simulink model "CRC"  (R2021a)
settings: Solver=ode45  StartTime=0.0  StopTime=10  RelTol=1e-3  EnableMultiTasking=on
model workspace (MAT data in the model file):
  frame_length = -4
undefined symbols (not defined in the file): CRC_degree
libraries: simulink x3, commcrc2 x2, dspswit3 x1
settings Model: Creator=student  LastModifiedBy=mitry
settings SolverCC: AlgebraicLoopSolver=TrustRegion
settings DataIOCC: LimitDataPoints=on  SaveFormat=Array  SignalLoggingSaveFormat=ModelDataLogs  ReturnWorkspaceOutputs=off
settings OptimizationCC: InitFltsAndDblsToZero=on  LifeSpan=inf
settings DebuggingCC: SaveWithParameterizedLinksMsg=none  UnderspecifiedInitializationDetection=Classic  MergeDetectMultiDrivingBlocksExec=none  SignalResolutionControl=TryResolveAllWithWarning  SolverPrmCheckMsg=warning  MultiTaskDSMMsg=warning  MultiTaskCondExecSysMsg=none  AllowSymbolicDim=off  SFUnexpectedBacktrackingDiag=warning  SFNoUnconditionalDefaultTransitionDiag=warning  SFExecutionAtInitializationDiag=none  SFMachineParentedDataDiag=warning  ArithmeticOperatorsInVariantConditions=warning
settings HardwareCC: ProdBitPerPointer=32  ProdBitPerSizeT=32  ProdBitPerPtrDiffT=32  ProdLargestAtomicFloat=None  ProdIntDivRoundTo=Undefined  ProdEndianess=Unspecified  ProdWordSize=32  ProdHWDeviceType=32-bit Generic
settings ModelReferenceCC: PropagateSignalLabelsOutOfModel=off
settings SFSimCC: SimUseLocalCustomCode=off  CustomCodeUndefinedFunction=UseInterfaceOnly
settings RTWCC: RTWUseLocalCustomCode=off
settings CodeAppCC: StateflowObjectComments=on
settings GRTTargetCC: TargetFcnLib=ansi_tfl_tmw.mat  TargetLangStandard=C89/C90 (ANSI)  CombineOutputUpdateFcns=off  GRTInterface=on
settings ConfigComp: CovMetricSettings=dw  CovSaveCumulativeToWorkspaceVar=on  CovSaveSingleToWorkspaceVar=on  CovExternalEMLEnable=off

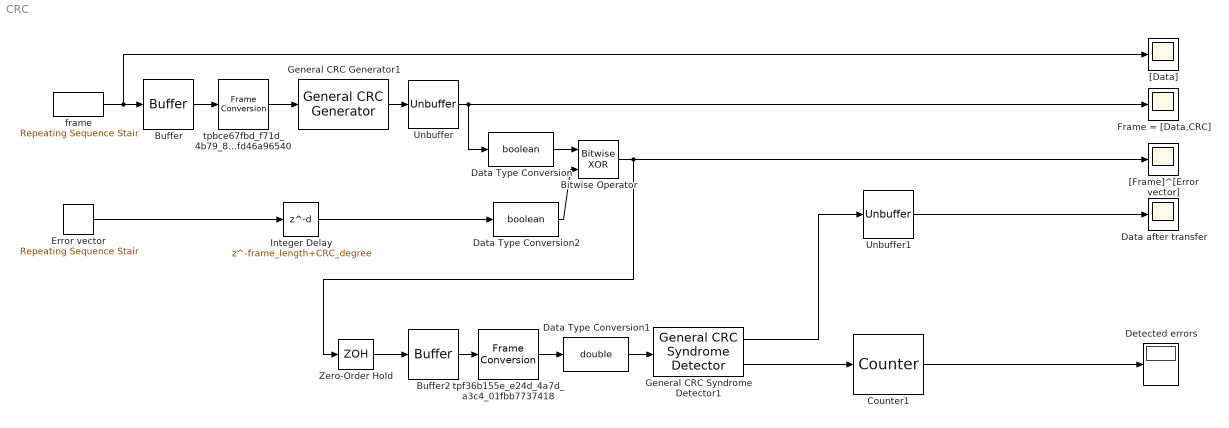
== system CRC ==
  Bitwise Operator : simulink/Logic and Bit Operations/Bitwise Operator  logicop=XOR  UseBitMask=off  NumInputPorts=2  BitMask=bin2dec('11011001')  BitMaskRealWorld=Stored Integer
  Buffer : Buffer  N=frame_length  OutputFrames=off
  Buffer2 : Buffer  N=frame_length + CRC_degree  OutputFrames=off
  Counter1 : dspswit3/Counter  Direction=Up  CountEvent=Non-zero sample  CounterSize=User defined  MaxCount=65535  InitialCount=0  Output=Count  HitValue=32  ResetInput=off  SamplesPerFrame=1  Ts=1  CntDtype=double  HitDtype=Logical
  Data Type Conversion : DataTypeConversion  OutDataTypeStr=boolean
  Data Type Conversion1 : DataTypeConversion  OutDataTypeStr=double
  Data Type Conversion2 : DataTypeConversion  OutDataTypeStr=boolean
  Data after transfer : Scope
  Detected errors : Display
      settings: Format=binary (Stored Integer)
  Error vector : simulink/Sources/Repeating Sequence Stair  OutValues=[0 0 0 0 0 0 0 0 0 0 0]  tsamp=1/(frame_length+CRC_degree)  OutMin=[]  OutMax=[]  OutDataTypeStr=float('double')  OutputDataTypeScalingMode=Specify via dialog  OutDataType=float('double')  ConRadixGroup=Best Precision: Vector-wise  OutScaling=2^-12
  Frame = [Data,CRC] : Scope
  General CRC Generator1 : commcrc2/General CRC Generator  genPoly=[1 0 1 1]  iniStates=[0]  directMethod=off  reflectInputBytes=off  reflectChecksums=off  finalXOR=0  numChecksums=1
      settings: SourceProductBaseCode=CM
  General CRC Syndrome Detector1 : commcrc2/General CRC Syndrome Detector  genPoly=[1 0 1 1]  iniStates=[0]  directMethod=off  reflectInputBytes=off  reflectChecksums=off  finalXOR=0  numChecksums=1
      settings: SourceProductBaseCode=CM
  Integer Delay : Delay  DelayLength=frame_length+CRC_degree  SampleTime=1/(frame_length+CRC_degree)
  Unbuffer : Unbuffer
  Unbuffer1 : Unbuffer
  Zero-Order Hold : ZeroOrderHold  SampleTime=1/(frame_length+CRC_degree)
  "[Data]" : Scope
  "[Frame]^[Error vector]" : Scope
  frame : simulink/Sources/Repeating Sequence Stair  OutValues=[1 0 1 1 1 0 0 1]  tsamp=1/frame_length  OutMin=[]  OutMax=[]  OutDataTypeStr=float('double')  OutputDataTypeScalingMode=Specify via dialog  OutDataType=float('double')  ConRadixGroup=Use specified scaling  OutScaling=2^8
  tpbce67fbd_f71d_4b79_8b88_b9fd46a96540 : FrameConversion
  tpf36b155e_e24d_4a7d_a3c4_01fbb7737418 : FrameConversion
  wires:
  Unbuffer/1 -> Data Type Conversion/1, Frame = [Data,CRC]/1
  General CRC Generator1/1 -> Unbuffer/1
  Unbuffer1/1 -> Data after transfer/1
  General CRC Syndrome Detector1/1 -> Unbuffer1/1
  Error vector/1 -> Integer Delay/1
  Data Type Conversion/1 -> Bitwise Operator/1
  Data Type Conversion1/1 -> General CRC Syndrome Detector1/1
  Data Type Conversion2/1 -> Bitwise Operator/2
  General CRC Syndrome Detector1/2 -> Counter1/1
  Bitwise Operator/1 -> Zero-Order Hold/1, "[Frame]^[Error vector]"/1
  Integer Delay/1 -> Data Type Conversion2/1
  frame/1 -> Buffer/1, "[Data]"/1
  Zero-Order Hold/1 -> Buffer2/1
  Counter1/1 -> Detected errors/1
  Buffer/1 -> tpbce67fbd_f71d_4b79_8b88_b9fd46a96540/1
  tpbce67fbd_f71d_4b79_8b88_b9fd46a96540/1 -> General CRC Generator1/1
  Buffer2/1 -> tpf36b155e_e24d_4a7d_a3c4_01fbb7737418/1
  tpf36b155e_e24d_4a7d_a3c4_01fbb7737418/1 -> Data Type Conversion1/1
